simulink model "heli_quanser_base_MC"  (R2025a)
settings: Solver=FixedStepAuto  StartTime=0.0  StopTime=5  FixedStep=0.001  RelTol=1e-3  EnableMultiTasking=on
values from neighbouring files (symbols this model uses):
  Ts = 1    [heli_ls_ident.m]    (also in minimos_cuadrados.m)
undefined symbols (not defined in the file or in its folder): B_p, B_y, g, J_eq_p, J_eq_y, K_pp, K_py, K_yp, K_yy, l_cm, m_heli, theta_0, VMAX_UPM_P, VMAX_UPM_Y
libraries: simulink x2, simulink_extras x1
settings Model: Creator=Jorge Romero  LastModifiedBy=440G5
settings SolverCC: AlgebraicLoopSolver=TrustRegion
settings DataIOCC: LimitDataPoints=on  SaveFormat=Array  ReturnWorkspaceOutputs=off
settings OptimizationCC: ExpressionDepthLimit=2147483647.0  LifeSpan=inf
settings DebuggingCC: UnderspecifiedInitializationDetection=Classic  MergeDetectMultiDrivingBlocksExec=none  SolverPrmCheckMsg=warning  UnconnectedInputMsg=warning  UnconnectedOutputMsg=warning  UnconnectedLineMsg=warning  StateNameClashWarn=warning  SFUnexpectedBacktrackingDiag=warning  SFNoUnconditionalDefaultTransitionDiag=warning  SFExecutionAtInitializationDiag=none  ArithmeticOperatorsInVariantConditions=warning
settings HardwareCC: ProdBitPerPointer=32.0  ProdBitPerSizeT=32.0  ProdBitPerPtrDiffT=32.0  ProdLargestAtomicFloat=None  ProdIntDivRoundTo=Undefined  ProdEndianess=Unspecified  ProdWordSize=32.0  ProdHWDeviceType=32-bit Generic
settings ModelReferenceCC: EnableRefExpFcnMdlSchedulingChecks=on  PropagateSignalLabelsOutOfModel=off
settings SFSimCC: SimUseLocalCustomCode=off  CustomCodeUndefinedFunction=UseInterfaceOnly
settings RTWCC: RTWUseLocalCustomCode=off  GPUComputeCapability=3.5  DLArmComputeVersion=19.05
settings CodeAppCC: StateflowObjectComments=on
settings GRTTargetCC: TargetLangStandard=C89/C90 (ANSI)
settings ConfigComp: CovMetricSettings=dw  CovSaveCumulativeToWorkspaceVar=on  CovSaveSingleToWorkspaceVar=on  CovExternalEMLEnable=off

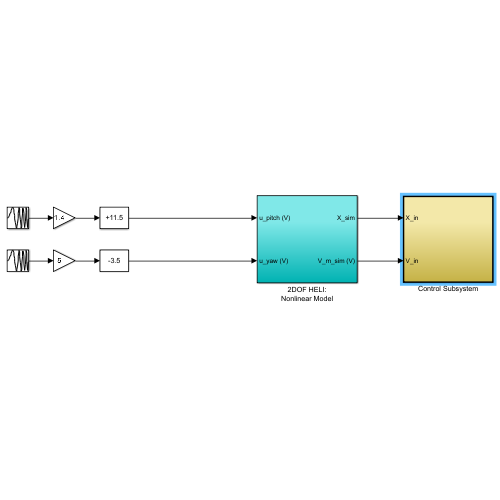
[thumbnail: Simulink's stored preview of the top-level diagram]
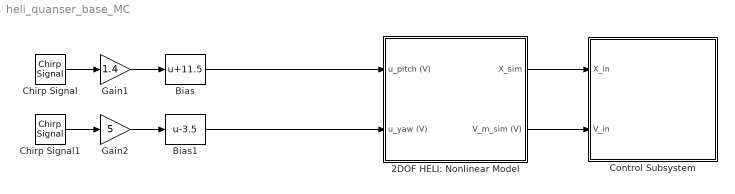
== system heli_quanser_base_MC ==
  2DOF HELI: Nonlinear Model : Subsystem
  Bias : Bias  Bias=11.5  SaturateOnIntegerOverflow=off
  Bias1 : Bias  Bias=-3.5  SaturateOnIntegerOverflow=off
  Chirp Signal : simulink/Sources/Chirp Signal  f1=0.08  T=10  f2=1
  Chirp Signal1 : simulink/Sources/Chirp Signal  f1=0.05  T=100  f2=1
  Control Subsystem : Subsystem  TreatAsAtomicUnit=on
  Gain1 : Gain  Gain=1.4
  Gain2 : Gain  Gain=5
  wires:
  Gain2/1 -> Bias1/1
  Gain1/1 -> Bias/1
  Chirp Signal1/1 -> Gain2/1
  Chirp Signal/1 -> Gain1/1
  Bias/1 -> 2DOF HELI: Nonlinear Model/1(u_pitch (V))
  Bias1/1 -> 2DOF HELI: Nonlinear Model/2(u_yaw (V))
  2DOF HELI: Nonlinear Model/1(X_sim) -> Control Subsystem/1(X_in)
  2DOF HELI: Nonlinear Model/2(V_m_sim (V)) -> Control Subsystem/2(V_in)

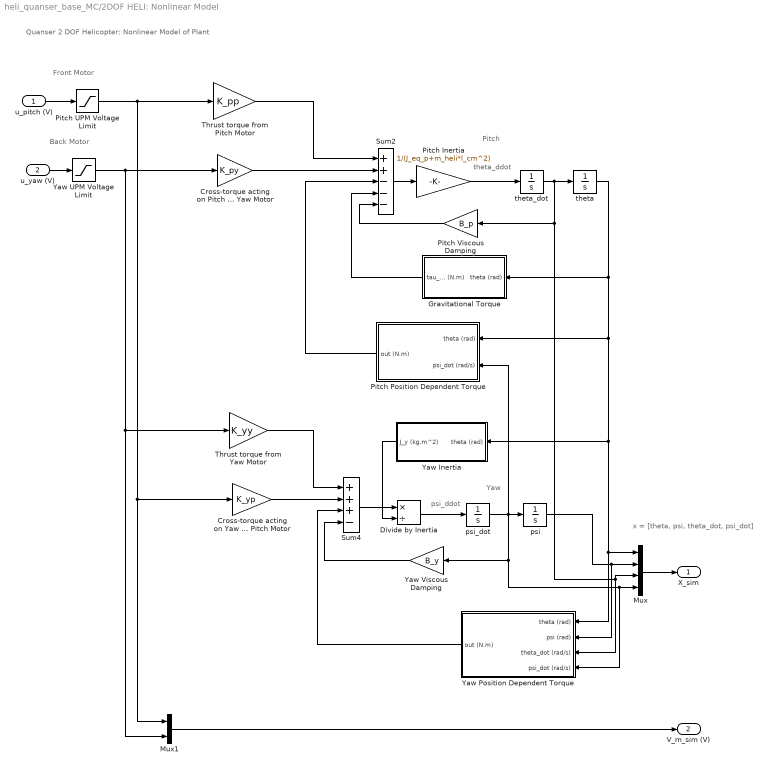
== system heli_quanser_base_MC/2DOF HELI: Nonlinear Model ==
  note: Back Motor
  note: Front Motor
  note: x = [theta, psi, theta_dot, psi_dot]
  note: Quanser 2 DOF Helicopter: Nonlinear Model of Plant
  note: theta_ddot
  note: psi_ddot
  note: Pitch
  note: Yaw
  u_pitch (V) : Inport
  u_yaw (V) : Inport  Port=2
  Cross-torque acting on Pitch from Yaw Motor : Gain  Gain=K_py
  Cross-torque acting on Yaw from Pitch Motor : Gain  Gain=K_yp
  Divide by Inertia : Product  Inputs=*/
  Gravitational Torque : Subsystem
  Mux : Mux
  Mux1 : Mux  Inputs=2
  Pitch Inertia : Gain  Gain=1/(J_eq_p+m_heli*l_cm^2)
  Pitch Position Dependent Torque : Subsystem  AncestorBlock=heli_2d_lib/2DOF Helicopter: Nonlinear Model/Yaw Nonlinear Element
  Pitch UPM Voltage Limit : Saturate  UpperLimit=VMAX_UPM_P  LowerLimit=- VMAX_UPM_P
  Pitch Viscous Damping : Gain  Gain=B_p
  Sum2 : Sum  Inputs=++---
  Sum4 : Sum  Inputs=+++-
  Thrust torque from Pitch Motor : Gain  Gain=K_pp
  Thrust torque from Yaw Motor : Gain  Gain=K_yy
  Yaw Inertia : Subsystem
  Yaw Position Dependent Torque : Subsystem
  Yaw UPM Voltage Limit : Saturate  UpperLimit=VMAX_UPM_Y  LowerLimit=- VMAX_UPM_Y
  Yaw Viscous Damping : Gain  Gain=B_y
  psi : Integrator
  psi_dot : Integrator
  theta : Integrator  InitialCondition=theta_0  LimitOutput=on  UpperSaturationLimit=40.5*pi/180  LowerSaturationLimit=-40.5*pi/180
  theta_dot : Integrator
  X_sim : Outport
  V_m_sim (V) : Outport  Port=2
  wires:
  Pitch Position Dependent Torque/1(out (N.m)) -> Sum2/3
  Gravitational Torque/1(tau_g (N.m)) -> Sum2/4
  Pitch Viscous Damping/1 -> Sum2/5
  Cross-torque acting on Pitch from Yaw Motor/1 -> Sum2/2
  Thrust torque from Pitch Motor/1 -> Sum2/1
  Yaw Inertia/1(J_y (kg.m^2)) -> Divide by Inertia/2
  Divide by Inertia/1 -> psi_dot/1
  Sum4/1 -> Divide by Inertia/1
  Yaw Position Dependent Torque/1(out (N.m)) -> Sum4/3
  Yaw Viscous Damping/1 -> Sum4/4
  psi/1 -> Yaw Position Dependent Torque/2(psi (rad)), Mux/2
  Mux1/1 -> V_m_sim (V)/1
  Yaw UPM Voltage Limit/1 -> Thrust torque from Yaw Motor/1, Mux1/2, Cross-torque acting on Pitch from Yaw Motor/1
  Pitch UPM Voltage Limit/1 -> Mux1/1, Cross-torque acting on Yaw from Pitch Motor/1, Thrust torque from Pitch Motor/1
  Mux/1 -> X_sim/1
  theta/1 -> Gravitational Torque/1(theta (rad)), Pitch Position Dependent Torque/1(theta (rad)), Yaw Position Dependent Torque/1(theta (rad)), Mux/1, Yaw Inertia/1(theta (rad))
  Sum2/1 -> Pitch Inertia/1
  Pitch Inertia/1 -> theta_dot/1
  theta_dot/1 -> Pitch Viscous Damping/1, Yaw Position Dependent Torque/3(theta_dot (rad/s)), Mux/3, theta/1
  Thrust torque from Yaw Motor/1 -> Sum4/1
  Cross-torque acting on Yaw from Pitch Motor/1 -> Sum4/2
  psi_dot/1 -> Yaw Viscous Damping/1, Yaw Position Dependent Torque/4(psi_dot (rad/s)), Mux/4, Pitch Position Dependent Torque/2(psi_dot (rad/s)), psi/1
  u_pitch (V)/1 -> Pitch UPM Voltage Limit/1
  u_yaw (V)/1 -> Yaw UPM Voltage Limit/1

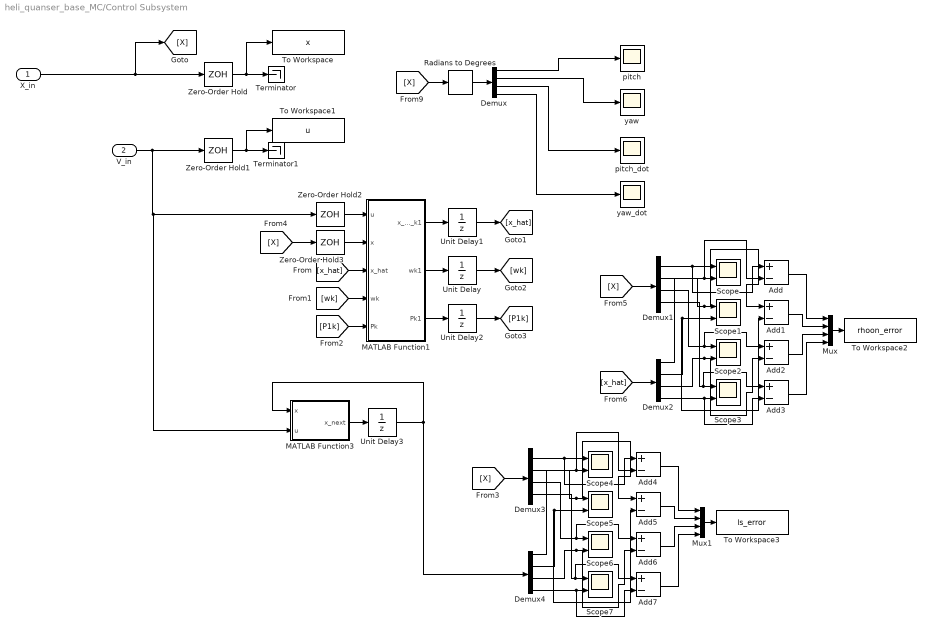
== system heli_quanser_base_MC/Control Subsystem ==
  X_in : Inport
  V_in : Inport  Port=2
  Add{,1..7} (8 alike) : Sum  Inputs=+-
  Demux{,1..4} (5 alike) : Demux
      Demux settings: DisplayOption=none
  MATLAB Function1 : MATLAB Function  TreatAsAtomicUnit=on
  MATLAB Function3 : MATLAB Function  TreatAsAtomicUnit=on
  Mux : Mux
  Mux1 : Mux
  Radians to Degrees : simulink_extras/Transformations/Radians to Degrees
  Scope{,1..7} (8 alike) : Scope  NumInputPorts=2
      Scope settings: ActiveDisplayYMinimum=-1.1415026108241673  ActiveDisplayYMaximum=0.12683362342490745  DataLoggingVariableName=ScopeData4
      Scope1 settings: ActiveDisplayYMinimum=0.00065987107501674913  ActiveDisplayYMaximum=4.6512841717291593  DataLoggingVariableName=ScopeData5
      Scope2 settings: ActiveDisplayYMinimum=-136.21614176214669  ActiveDisplayYMaximum=1171.9792706431781  DataLoggingVariableName=ScopeData6
      Scope3 settings: ActiveDisplayYMinimum=-1.1741616508954156  ActiveDisplayYMaximum=1.4302738530662835  DataLoggingVariableName=ScopeData7
      Scope4 settings: ActiveDisplayYMinimum=-0.78569456230161683  ActiveDisplayYMaximum=0.0026675901375168704  DataLoggingVariableName=ScopeData8
      Scope5 settings: ActiveDisplayYMinimum=-0.45463938909370377  ActiveDisplayYMaximum=4.0917545018433348  DataLoggingVariableName=ScopeData9
      Scope6 settings: ActiveDisplayYMinimum=-0.49237684754972044  ActiveDisplayYMaximum=0.55901528153260716  DataLoggingVariableName=ScopeData10
      Scope7 settings: ActiveDisplayYMinimum=-0.14622878783376417  ActiveDisplayYMaximum=1.3160590905038778  DataLoggingVariableName=ScopeData11
  Terminator : Terminator
  Terminator1 : Terminator
  To Workspace : ToWorkspace  VariableName=x  SaveFormat=Timeseries  SampleTime=-1
  To Workspace1 : ToWorkspace  VariableName=u  SaveFormat=Timeseries  SampleTime=-1
  To Workspace2 : ToWorkspace  VariableName=rhoon_error  SaveFormat=Timeseries  SampleTime=-1
  To Workspace3 : ToWorkspace  VariableName=ls_error  SaveFormat=Timeseries  SampleTime=-1
  Unit Delay : UnitDelay  InitialCondition=rand(16,1)  SampleTime=-1  HasFrameUpgradeWarning=on
  Unit Delay1 : UnitDelay  SampleTime=-1  HasFrameUpgradeWarning=on
  Unit Delay2 : UnitDelay  InitialCondition=repmat(5e4*eye(4), [1 1 4])  SampleTime=-1  HasFrameUpgradeWarning=on
  Unit Delay3 : UnitDelay  InitialCondition=|  SampleTime=-1  HasFrameUpgradeWarning=on
      | [ -40.5*pi/180 ;
      |         0 ;
      |         0 ;
      |         0 ];
  Zero-Order Hold2 : ZeroOrderHold  SampleTime=-1
  Zero-Order Hold3 : ZeroOrderHold  SampleTime=-1
  Zero-Order Hold : ZeroOrderHold  SampleTime=Ts
  Zero-Order Hold1 : ZeroOrderHold  SampleTime=Ts
  pitch : Scope
      settings: TimeSpan=30  ActiveDisplayYMinimum=-81.99762  ActiveDisplayYMaximum=9.11085
  pitch_dot : Scope
      settings: TimeSpan=30  ActiveDisplayYMinimum=-48.65452  ActiveDisplayYMaximum=62.46494
  yaw : Scope
      settings: TimeSpan=30  ActiveDisplayYMinimum=-31.83031  ActiveDisplayYMaximum=286.47281  DataLoggingVariableName=ScopeData2
  yaw_dot : Scope
      settings: TimeSpan=30  ActiveDisplayYMinimum=-83.27416  ActiveDisplayYMaximum=83.72639  DataLoggingVariableName=ScopeData3
  wires:
  Demux/1 -> pitch/1
  Demux/4 -> yaw_dot/1
  Radians to Degrees/1 -> Demux/1
  [X] -> Radians to Degrees/1
  Demux/3 -> pitch_dot/1
  Demux/2 -> yaw/1
  Zero-Order Hold/1 -> To Workspace/1, Terminator/1
  Zero-Order Hold1/1 -> To Workspace1/1, Terminator1/1
  [x_hat] -> MATLAB Function1/3(x_hat)
  Unit Delay1/1 -> [x_hat]
  MATLAB Function1/2(wk1) -> Unit Delay/1
  MATLAB Function1/3(Pk1) -> Unit Delay2/1
  Zero-Order Hold2/1 -> MATLAB Function1/1(u)
  Unit Delay2/1 -> [P1k]
  [P1k] -> MATLAB Function1/5(Pk)
  Unit Delay/1 -> [wk]
  MATLAB Function1/1(x_hat_k1) -> Unit Delay1/1
  Zero-Order Hold3/1 -> MATLAB Function1/2(x)
  [wk] -> MATLAB Function1/4(wk)
  V_in/1 -> MATLAB Function3/2(u), Zero-Order Hold2/1, Zero-Order Hold1/1
  [X] -> Zero-Order Hold3/1
  Demux1/3 -> Add2/1, Scope2/1
  Demux1/2 -> Add1/1, Scope1/1
  [x_hat] -> Demux2/1
  Demux2/2 -> Scope1/2, Add1/2
  Demux2/4 -> Add3/2, Scope3/2
  Demux2/1 -> Add/2, Scope/2
  [X] -> Demux1/1
  Demux1/1 -> Add/1, Scope/1
  Demux1/4 -> Add3/1, Scope3/1
  Demux2/3 -> Add2/2, Scope2/2
  X_in/1 -> [X], Zero-Order Hold/1
  Add/1 -> Mux/1
  Add1/1 -> Mux/2
  Add2/1 -> Mux/3
  Add3/1 -> Mux/4
  Mux/1 -> To Workspace2/1
  MATLAB Function3/1(x_next) -> Unit Delay3/1
  Add6/1 -> Mux1/3
  Add4/1 -> Mux1/1
  Demux4/4 -> Add7/2, Scope7/2
  [X] -> Demux3/1
  Demux3/1 -> Add4/1, Scope4/1
  Demux3/4 -> Add7/1, Scope7/1
  Demux3/2 -> Add5/1, Scope5/1
  Mux1/1 -> To Workspace3/1
  Add7/1 -> Mux1/4
  Demux3/3 -> Add6/1, Scope6/1
  Add5/1 -> Mux1/2
  Demux4/3 -> Add6/2, Scope6/2
  Demux4/2 -> Scope5/2, Add5/2
  Unit Delay3/1 -> Demux4/1, MATLAB Function3/1(x)
  Demux4/1 -> Add4/2, Scope4/2

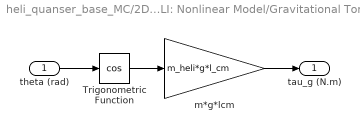
== system heli_quanser_base_MC/2DOF HELI: Nonlinear Model/Gravitational Torque ==
  theta (rad) : Inport
  Trigonometric Function : Trigonometry  Operator=cos  OutputSignalType=real
  m*g*lcm : Gain  Gain=m_heli*g*l_cm
  tau_g (N.m) : Outport
  wires:
  m*g*lcm/1 -> tau_g (N.m)/1
  theta (rad)/1 -> Trigonometric Function/1
  Trigonometric Function/1 -> m*g*lcm/1

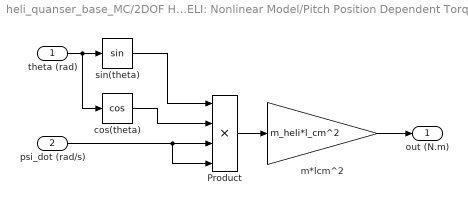
== system heli_quanser_base_MC/2DOF HELI: Nonlinear Model/Pitch Position Dependent Torque ==
  theta (rad) : Inport
  psi_dot (rad/s) : Inport  Port=2
  Product : Product  Inputs=4  RndMeth=Zero
  cos(theta) : Trigonometry  Operator=cos  OutputSignalType=real
  m*lcm^2 : Gain  Gain=m_heli*l_cm^2
  sin(theta) : Trigonometry  OutputSignalType=real
  out (N.m) : Outport
  wires:
  psi_dot (rad/s)/1 -> Product/4, Product/3
  theta (rad)/1 -> cos(theta)/1, sin(theta)/1
  Product/1 -> m*lcm^2/1
  sin(theta)/1 -> Product/1
  cos(theta)/1 -> Product/2
  m*lcm^2/1 -> out (N.m)/1

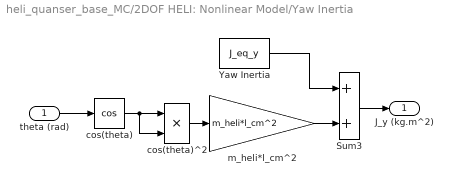
== system heli_quanser_base_MC/2DOF HELI: Nonlinear Model/Yaw Inertia ==
  theta (rad) : Inport
  Sum3 : Sum
  Yaw Inertia : Constant  Value=J_eq_y
  cos(theta) : Trigonometry  Operator=cos  OutputSignalType=real
  cos(theta)^2 : Product  RndMeth=Zero
  m_heli*l_cm^2 : Gain  Gain=m_heli*l_cm^2
  J_y (kg.m^2) : Outport
  wires:
  cos(theta)/1 -> cos(theta)^2/2, cos(theta)^2/1
  Sum3/1 -> J_y (kg.m^2)/1
  theta (rad)/1 -> cos(theta)/1
  m_heli*l_cm^2/1 -> Sum3/2
  Yaw Inertia/1 -> Sum3/1
  cos(theta)^2/1 -> m_heli*l_cm^2/1

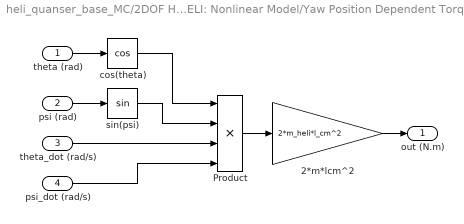
== system heli_quanser_base_MC/2DOF HELI: Nonlinear Model/Yaw Position Dependent Torque ==
  theta (rad) : Inport
  psi (rad) : Inport  Port=2
  theta_dot (rad/s) : Inport  Port=3
  psi_dot (rad/s) : Inport  Port=4
  2*m*lcm^2 : Gain  Gain=2*m_heli*l_cm^2
  Product : Product  Inputs=4  RndMeth=Zero
  cos(theta) : Trigonometry  Operator=cos  OutputSignalType=real
  sin(psi) : Trigonometry  OutputSignalType=real
  out (N.m) : Outport
  wires:
  2*m*lcm^2/1 -> out (N.m)/1
  psi_dot (rad/s)/1 -> Product/4
  theta_dot (rad/s)/1 -> Product/3
  sin(psi)/1 -> Product/2
  cos(theta)/1 -> Product/1
  Product/1 -> 2*m*lcm^2/1
  theta (rad)/1 -> cos(theta)/1
  psi (rad)/1 -> sin(psi)/1

== matlab function heli_quanser_base_MC/Control Subsystem/MATLAB Function1 ==
  data: u input; x input; x_hat input; wk input; Pk input; x_hat_k1 output; wk1 output; Pk1 output
function [x_hat_k1, wk1, Pk1] = rhonn_rotary(u, x, x_hat, wk, Pk)
% RHONN para péndulo rotatorio (Furuta) con 4 estados:
% x = [beta; betadot; gamma; gammadot]
%
% Entradas:
%   u    : vector de entrada [2x1] (p. ej., dos torques o dos señales)
%   x    : vector de estado medido [4x1]
%   x_hat: estimación actual del estado [4x1]
%   wk   : vector de pesos [16x1] ordenado por estado (4 pesos por estado)
%   Pk   : matrices de covarianza por estado [4x4x4]
%
% Salidas:
%   x_hat_k1 : predicción neuronal del estado siguiente [4x1]
%   wk1      : pesos actualizados [16x1]
%   Pk1      : covarianzas actualizadas [4x4x4]

%% Comprobaciones rápidas de tamaño (opcional pero útil)
if ~isequal(size(u), [2,1])
    error('u debe ser [2x1]. Recibido %s.', mat2str(size(u)));
end
if ~isequal(size(x), [4,1]) || ~isequal(size(x_hat), [4,1])
    error('x y x_hat deben ser [4x1].');
end
if ~isequal(size(wk), [16,1])
    error('wk debe ser [16x1].');
end
if ~isequal(size(Pk), [4,4,4])
    error('Pk debe ser [4x4x4].');
end

%% Ganancias fijas de entrada (ahora vectores 2x1)
% Ajusta estos valores a tu planta/escala:
w_u2 = [0.15; 0.00];   % contribución de u a x2 (betadot)
w_u4 = [0.00; 0.15];   % contribución de u a x4 (gammadot)
% Nota: si ambos actuadores afectan ambos estados, pon valores no nulos en ambas posiciones.

%% Extrae pesos por estado (cada w_i es [4x1])
w1 = wk( 1: 4);   % para x1 (beta)
w2 = wk( 5: 8);   % para x2 (betadot)
w3 = wk( 9:12);   % para x3 (gamma)
w4 = wk(13:16);   % para x4 (gammadot)

%% Vector de regresores no lineales (H: [4x1])
H = [tanh(x(1));
     tanh(x(2));
     tanh(x(3));
     tanh(x(4))];

%% Predicción neuronal (modelo RHONN)
x1_hat = w1.'*H;                  % beta
x2_hat = w2.'*H + w_u2.'*u;       % betadot  (+ entrada 2x1)
x3_hat = w3.'*H;                  % gamma
x4_hat = w4.'*H + w_u4.'*u;       % gammadot (+ entrada 2x1)

x_hat_k1 = [x1_hat; x2_hat; x3_hat; x4_hat];

%% EKF por estado (lineal en parámetros con respecto a H)
Q = eye(4)*5e3;   % proceso en espacio de pesos
R = 6e3;          % varianza de medición (escalar por estado)

Pk1 = Pk;         % preasigna
wk1 = wk;         % preasigna

% Error con respecto a la estimación actual
e = x - x_hat;    % [4x1]

% ---- Estado 1 ----
P1 = Pk(:,:,1);
K1 = (P1*H) / (R + H.'*P1*H);
w1_new = w1 + K1 * e(1);
P1_new = P1 - K1*(H.')*P1 + Q;

% ---- Estado 2 ----
P2 = Pk(:,:,2);
K2 = (P2*H) / (R + H.'*P2*H);
w2_new = w2 + K2 * e(2);
P2_new = P2 - K2*(H.')*P2 + Q;

% ---- Estado 3 ----
P3 = Pk(:,:,3);
K3 = (P3*H) / (R + H.'*P3*H);
w3_new = w3 + K3 * e(3);
P3_new = P3 - K3*(H.')*P3 + Q;

% ---- Estado 4 ----
P4 = Pk(:,:,4);
K4 = (P4*H) / (R + H.'*P4*H);
w4_new = w4 + K4 * e(4);
P4_new = P4 - K4*(H.')*P4 + Q;

%% Empaqueta resultados
wk1 = [w1_new; w2_new; w3_new; w4_new];
Pk1(:,:,1) = P1_new;
Pk1(:,:,2) = P2_new;
Pk1(:,:,3) = P3_new;
Pk1(:,:,4) = P4_new;
end

== matlab function heli_quanser_base_MC/Control Subsystem/MATLAB Function3 ==
  data: x input; u input; x_next output
function x_next = ss_disc_bias(x, u)
%#codegen
% Discrete state-space with bias:
%   x(k+1) = A*x(k) + B*u(k) + c
% Inputs:
%   x : [4x1] current state
%   u : [2x1] input
% Output:
%   x_next : [4x1] next state

% ----- matrices identificadas -----
A = [ 1.0000   -0.0000    0.0010    0.0000;
     -0.0000    1.0000    0.0000    0.0010;
     -0.0134   -0.0014    0.9912    0.0148;
     -0.0004   -0.0001    0.0002    0.9973 ];

B = [ 0.0000   -0.0000;
      0.0000    0.0000;
      0.0013   -0.0025;
      0.0003    0.0007 ];

c = [ -0.0000;
      -0.0000;
      -0.0281;
      -0.0012 ];

% ----- dinámica discreta -----
x_next = A * x + B * u + c;
end
